simulink model "TestSetup"  (R2022a)
settings: Solver=VariableStepAuto  StartTime=0.0  StopTime=10.0  RelTol=1e-3
undefined symbols (not defined in the file or in its folder): ignition_1, ignition_2, ignition_3, ignition_4, ignition_dwell_time, injection_duration, injection_start_1, injection_start_2, injection_start_3, injection_start_4
libraries: simulink x10
settings Model: Creator=feyzi  LastModifiedBy=feyzi

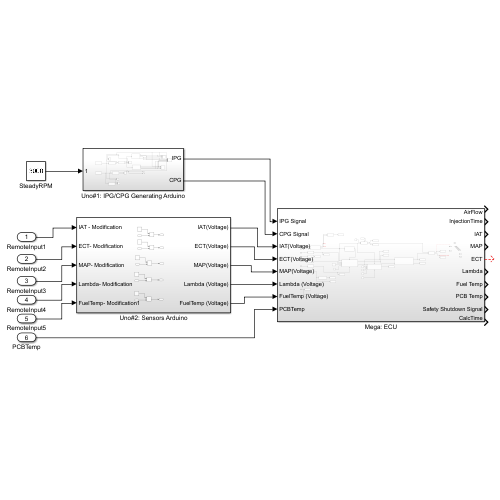
[thumbnail: Simulink's stored preview of the top-level diagram]
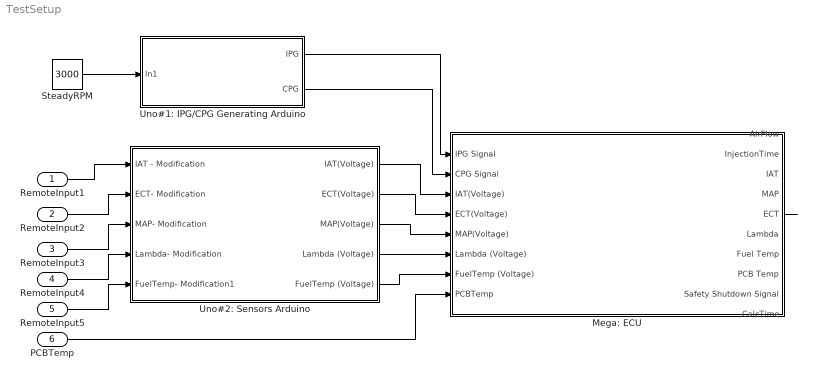
== system TestSetup ==
  RemoteInput1 : Inport
  RemoteInput2 : Inport  Port=2
  RemoteInput3 : Inport  Port=3
  RemoteInput4 : Inport  Port=4
  RemoteInput5 : Inport  Port=5
  PCBTemp : Inport  Port=6
  Mega: ECU : Subsystem
  SteadyRPM : Constant  Value=3000
  Uno#1: IPG/CPG Generating Arduino : Subsystem
  Uno#2: Sensors Arduino : Subsystem
  wires:
  RemoteInput1/1 -> Uno#2: Sensors Arduino/1(IAT - Modification)
  RemoteInput2/1 -> Uno#2: Sensors Arduino/2(ECT- Modification)
  RemoteInput3/1 -> Uno#2: Sensors Arduino/3(MAP- Modification)
  RemoteInput4/1 -> Uno#2: Sensors Arduino/4(Lambda- Modification)
  RemoteInput5/1 -> Uno#2: Sensors Arduino/5(FuelTemp- Modification1)
  Uno#2: Sensors Arduino/1(IAT(Voltage)) -> Mega: ECU/3(IAT(Voltage))
  Uno#2: Sensors Arduino/2(ECT(Voltage)) -> Mega: ECU/4(ECT(Voltage))
  Uno#2: Sensors Arduino/3(MAP(Voltage)) -> Mega: ECU/5(MAP(Voltage))
  Uno#2: Sensors Arduino/4(Lambda (Voltage)) -> Mega: ECU/6(Lambda (Voltage))
  Uno#2: Sensors Arduino/5(FuelTemp (Voltage)) -> Mega: ECU/7(FuelTemp (Voltage))
  PCBTemp/1 -> Mega: ECU/8(PCBTemp)
  SteadyRPM/1 -> Uno#1: IPG/CPG Generating Arduino/1(In1)
  Uno#1: IPG/CPG Generating Arduino/1(IPG) -> Mega: ECU/1(IPG Signal)
  Uno#1: IPG/CPG Generating Arduino/2(CPG) -> Mega: ECU/2(CPG Signal)
  Mega: ECU/5(ECT) -> ?

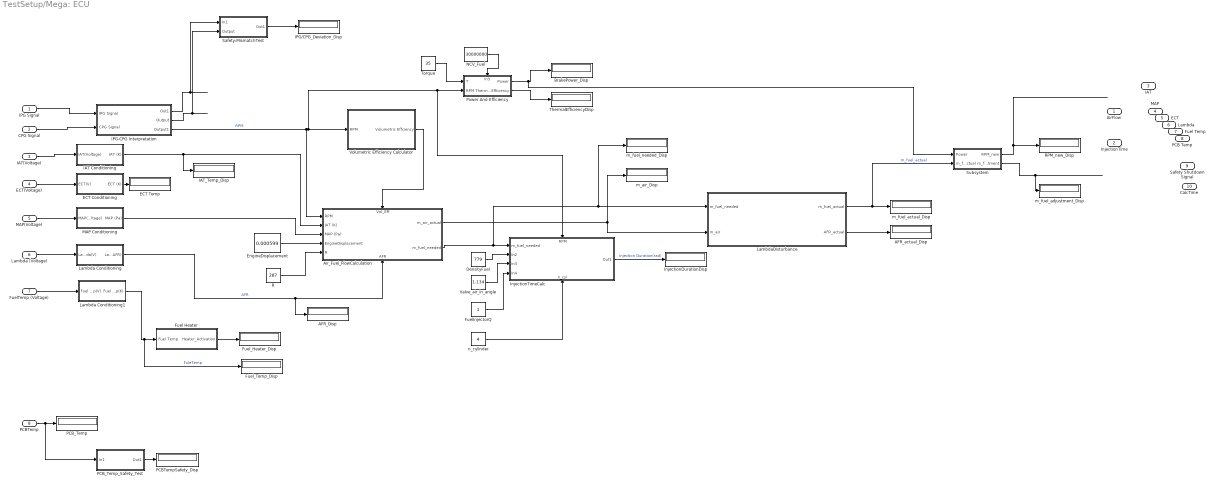
== system TestSetup/Mega: ECU ==
  IPG Signal : Inport
  CPG Signal : Inport  Port=2
  IAT(Voltage) : Inport  Port=3
  ECT(Voltage) : Inport  Port=4
  MAP(Voltage) : Inport  Port=5
  Lambda (Voltage) : Inport  Port=6
  FuelTemp (Voltage) : Inport  Port=7
  PCBTemp : Inport  Port=8
  AFR_Disp : Display
  AFR_actual_Disp : Display
  Air_Fuel_FlowCalculation : Subsystem
      settings: PortSchema="{\"entries\":[{\"content\":{\"sides\":[{\"content\":{\"connectorIds\":[\"In1\",\"In2\",\"In3\",\"In4\",\"In5\"]},\"type\":\"ConnectorPlacement.EquallySpacedRectSide\",\"uuid\":\"ac837b3a-3299-4579-a5f4-28e6eceafe2a\"},{\"content\":{\"connectorIds\":[\"Out1\",\"Out2\"],\"side\":\"RIGHT\"},\"type\":\"ConnectorPlacement.EquallySpacedRectSide\",\"uuid\":\"e1859a27-830c-4dac-bb73-ceffea8c29ce\"},{\"content\":{\"connectorIds\":[\"In6\"],\"side\":\"TOP\"},\"type\":\"ConnectorPlacement.EquallySpacedRectSide\",\"uuid\":\"f305f5bf-787a-4635-84c9-c02b37e24355\"},{\"content\":{\"connectorIds\":[\"In7\"],\"side\":\"BOTTOM\"},\"type\":\"ConnectorPlacement.EquallySpacedRectSide\",\"uuid\":\"b9c30ef4-a18f-4d96-bb00-033b4f03e588\"}]},\"type\":\"ConnectorPlacement.EquallySpacedConnector\",\"uuid\":\"e7c7efd2-9f43-49ae-a3b2-9ba67b40aa2d\"}],\"packageUris\":[\"http://schema.mathworks.com/mf0/Connector/R2020b\"],\"version\":\"1.0\"}"
  BrakePower_Disp : Display
  DensityFuel : Constant  Value=779
  ECT Conditioning : Subsystem
  ECT Temp : Display
  EngineDisplacement : Constant  Value=0.000599
  Fuel Heater : Subsystem
  FuelInjectorQ : Constant
  Fuel_Heater_Disp : Display
  Fuel_Temp_Disp : Display
  IAT Conditioning : Subsystem
  IAT_Temp_Disp : Display
  IPG-CPG Interpretation : Subsystem
  IPG/CPG_Deviation_Disp : Display
  InjectionDurationDisp : Display
  InjectionTimeCalc : Subsystem
      settings: PortSchema="{\"entries\":[{\"content\":{\"sides\":[{\"content\":{\"connectorIds\":[\"In1\",\"In2\",\"In3\",\"In4\"]},\"type\":\"ConnectorPlacement.EquallySpacedRectSide\",\"uuid\":\"ebdf0fa4-cc98-4ade-83ad-774b40e50e14\"},{\"content\":{\"connectorIds\":[\"Out1\"],\"side\":\"RIGHT\"},\"type\":\"ConnectorPlacement.EquallySpacedRectSide\",\"uuid\":\"8b1fcbdc-dea4-4525-97e7-1c674fd2a011\"},{\"content\":{\"connectorIds\":[\"In5\"],\"side\":\"TOP\"},\"type\":\"ConnectorPlacement.EquallySpacedRectSide\",\"uuid\":\"e38dc828-2b63-47c7-a128-8e05c6a6408b\"},{\"content\":{\"connectorIds\":[\"In6\"],\"side\":\"BOTTOM\"},\"type\":\"ConnectorPlacement.EquallySpacedRectSide\",\"uuid\":\"af069764-e087-4372-a960-1041a53fa6fc\"}]},\"type\":\"ConnectorPlacement.EquallySpacedConnector\",\"uuid\":\"8f444e95-b70b-4e07-afd3-af5c44a892f3\"}],\"packageUris\":[\"http://schema.mathworks.com/mf0/Connector/R2020b\"],\"version\":\"1.0\"}"
  Lambda Conditioning : Subsystem
  Lambda Conditioning1 : Subsystem
  LambdaDisturbance : Subsystem
  MAP Conditioning : Subsystem
  NCV_Fuel : Constant  Value=30000000
  PCBTempSafety_Disp : Display
  PCB_Temp : Display
  PCB_Temp_Safety_Test : Subsystem
  Power And Efficiency : Subsystem
      settings: PortSchema="{\"entries\":[{\"content\":{\"sides\":[{\"content\":{\"connectorIds\":[\"In1\",\"In2\"]},\"type\":\"ConnectorPlacement.EquallySpacedRectSide\",\"uuid\":\"acf79f69-6a10-44e4-b57d-bca1c6d4b241\"},{\"content\":{\"connectorIds\":[\"Out1\",\"Out2\"],\"side\":\"RIGHT\"},\"type\":\"ConnectorPlacement.EquallySpacedRectSide\",\"uuid\":\"336ed026-27e8-4de6-8253-c2a43c0fc710\"},{\"content\":{\"connectorIds\":[\"In3\"],\"side\":\"TOP\"},\"type\":\"ConnectorPlacement.EquallySpacedRectSide\",\"uuid\":\"3ecf9081-b2cf-495d-8221-6fb78c14c58c\"}]},\"type\":\"ConnectorPlacement.EquallySpacedConnector\",\"uuid\":\"3fda077c-3971-4965-af51-7420bd2b8db3\"}],\"packageUris\":[\"http://schema.mathworks.com/mf0/Connector/R2020b\"],\"version\":\"1.0\"}"
  R : Constant  Value=287
  RPM_new_Disp : Display
  Safety:MismatchTest : Subsystem
  Subsystem : Subsystem
  ThermalEfficiencyDisp : Display
  Torque : Constant  Value=35
  Valve_air_in_angle : Constant  Value=1.134
  Volumetric Efficiency Calculator : Subsystem
  m_air_Disp : Display
  m_fuel_actual_Disp : Display
  m_fuel_adjustment_Disp : Display
  m_fuel_needed_Disp : Display
  n_cylinder : Constant  Value=4
  AirFlow : Outport
  InjectionTime : Outport  Port=2
  IAT : Outport  Port=3
  MAP : Outport  Port=4
  ECT : Outport  Port=5
  Lambda : Outport  Port=6
  Fuel Temp : Outport  Port=7
  PCB Temp : Outport  Port=8
  Safety Shutdown Signal : Outport  Port=9
  CalcTime : Outport  Port=10
  wires:
  IPG Signal/1 -> IPG-CPG Interpretation/1(IPG Signal)
  CPG Signal/1 -> IPG-CPG Interpretation/2(CPG Signal)
  IPG-CPG Interpretation/1(Out1) -> Safety:MismatchTest/1(In1)
  IPG-CPG Interpretation/2(Output) -> Safety:MismatchTest/2(Output)
  ECT(Voltage)/1 -> ECT Conditioning/1(ECT(V))
  ECT Conditioning/1(ECT (K)) -> ECT Temp/1
  IAT(Voltage)/1 -> IAT Conditioning/1(IAT(Voltage))
  MAP(Voltage)/1 -> MAP Conditioning/1(MAP(Voltage))
  MAP Conditioning/1(MAP (Pa)) -> Air_Fuel_FlowCalculation/3(MAP (Pa))
  Lambda (Voltage)/1 -> Lambda Conditioning/1(Lambda(V))
  FuelTemp (Voltage)/1 -> Lambda Conditioning1/1(Fuel Temp(V))
  Volumetric Efficiency Calculator/1(Volumetric Effciency) -> Air_Fuel_FlowCalculation/6(Vol_Eff)
  EngineDisplacement/1 -> Air_Fuel_FlowCalculation/4(EngineDisplacement)
  R/1 -> Air_Fuel_FlowCalculation/5(R)
  IPG-CPG Interpretation/3(Output1) -> Air_Fuel_FlowCalculation/1(RPM), InjectionTimeCalc/5(RPM), Power And Efficiency/2(RPM), Volumetric Efficiency Calculator/1(RPM)  "RPM"
  IAT Conditioning/1(IAT (K)) -> IAT_Temp_Disp/1, Air_Fuel_FlowCalculation/2(IAT (K))
  Air_Fuel_FlowCalculation/1(m_air_actual) -> m_air_Disp/1, LambdaDisturbance/2(m_air)
  Torque/1 -> Power And Efficiency/1(T)
  Lambda Conditioning1/1(Fuel Temp(K)) -> Fuel_Temp_Disp/1, Fuel Heater/1(Fuel Temp)  "FuleTemp"
  Fuel Heater/1(Heater_Activation) -> Fuel_Heater_Disp/1
  Lambda Conditioning/1(Lambda(AFR)) -> AFR_Disp/1, Air_Fuel_FlowCalculation/7(AFR)  "AFR"
  Air_Fuel_FlowCalculation/2(m_fuel_needed) -> m_fuel_needed_Disp/1, LambdaDisturbance/1(m_fuel_needed), InjectionTimeCalc/1(m_fuel_needed)
  DensityFuel/1 -> InjectionTimeCalc/2(In2)
  Valve_air_in_angle/1 -> InjectionTimeCalc/3(In3)
  NCV_Fuel/1 -> Power And Efficiency/3(In3)
  FuelInjectorQ/1 -> InjectionTimeCalc/4(In4)
  InjectionTimeCalc/1(Out1) -> InjectionDurationDisp/1  "Injection Duration(rad)"
  LambdaDisturbance/1(m_fuel_actual) -> Subsystem/2(m_fuel_actual), m_fuel_actual_Disp/1  "m_fuel_actual"
  LambdaDisturbance/2(AFR_actual) -> AFR_actual_Disp/1
  Power And Efficiency/1(Power) -> Subsystem/1(Power), BrakePower_Disp/1
  Power And Efficiency/2(ThermalEfficiency) -> ThermalEfficiencyDisp/1
  n_cylinder/1 -> InjectionTimeCalc/6(n_cyl)
  Subsystem/1(RPM_new) -> RPM_new_Disp/1
  Subsystem/2(m_fuel_adjustment) -> m_fuel_adjustment_Disp/1
  Safety:MismatchTest/1(Out1) -> IPG/CPG_Deviation_Disp/1
  PCBTemp/1 -> PCB_Temp_Safety_Test/1(In1), PCB_Temp/1
  PCB_Temp_Safety_Test/1(Out1) -> PCBTempSafety_Disp/1

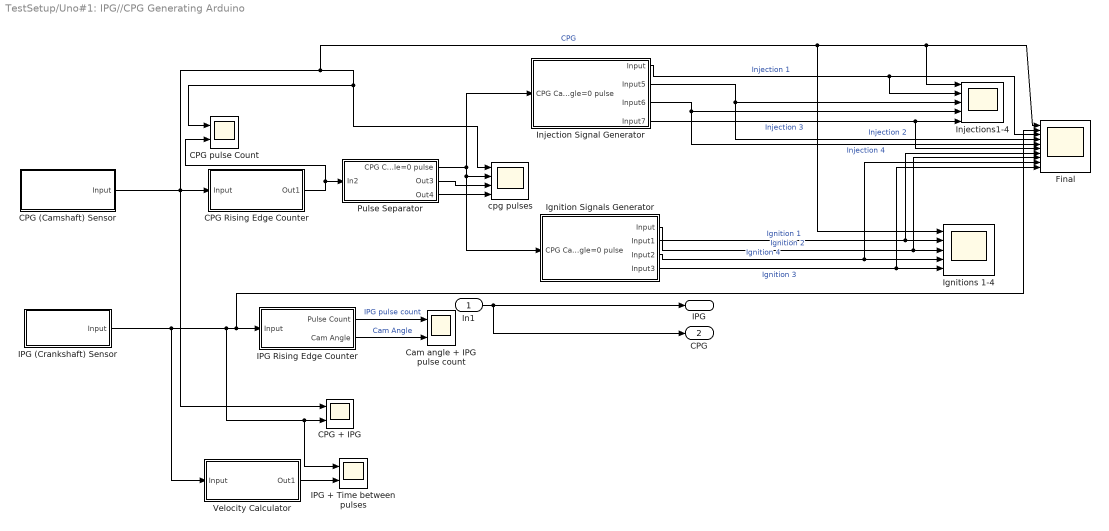
== system TestSetup/Uno#1: IPG//CPG Generating Arduino ==
  In1 : Inport
  CPG (Camshaft) Sensor : Subsystem
  CPG + IPG : Scope  NumInputPorts=2
  CPG Rising Edge Counter : Subsystem
  CPG pulse Count : Scope  NumInputPorts=2
  Cam angle + IPG pulse count : Scope  NumInputPorts=2
  Final : Scope  NumInputPorts=10
  IPG (Crankshaft) Sensor : Subsystem
  IPG + Time between pulses : Scope  NumInputPorts=2
  IPG Rising Edge Counter : Subsystem
  Ignition Signals Generator : Subsystem
  Ignitions 1-4 : Scope  NumInputPorts=5
  Injection Signal Generator : Subsystem
  Injections1-4 : Scope  NumInputPorts=5
  Pulse Separator : Subsystem
  Velocity Calculator : Subsystem
  cpg pulses : Scope  NumInputPorts=4
  IPG : Outport
  CPG : Outport  Port=2
  wires:
  In1/1 -> CPG/1, IPG/1
  IPG Rising Edge Counter/2(Cam Angle) -> Cam angle + IPG pulse count/2  "Cam Angle"
  IPG Rising Edge Counter/1(Pulse Count) -> Cam angle + IPG pulse count/1  "IPG pulse count"
  CPG Rising Edge Counter/1(Out1) -> Pulse Separator/1(In2), CPG pulse Count/2
  Velocity Calculator/1(Out1) -> IPG + Time between pulses/2
  Injection Signal Generator/1(Input) -> Injections1-4/2, Final/3  "Injection 1"
  Ignition Signals Generator/3(Input2) -> Final/9, Ignitions 1-4/4  "Ignition 4"
  Ignition Signals Generator/2(Input1) -> Final/8, Ignitions 1-4/3  "Ignition 2"
  Ignition Signals Generator/1(Input) -> Final/7, Ignitions 1-4/2  "Ignition 1"
  Injection Signal Generator/3(Input6) -> Final/5, Injections1-4/4  "Injection 4"
  Ignition Signals Generator/4(Input3) -> Final/10, Ignitions 1-4/5  "Ignition 3"
  IPG (Crankshaft) Sensor/1(Input) -> IPG Rising Edge Counter/1(Input), Final/2, CPG + IPG/2, IPG + Time between pulses/1, Velocity Calculator/1(Input)
  CPG (Camshaft) Sensor/1(Input) -> Final/1, Injections1-4/1, Ignitions 1-4/1, cpg pulses/1, CPG pulse Count/1, CPG Rising Edge Counter/1(Input), CPG + IPG/1  "CPG"
  Injection Signal Generator/4(Input7) -> Injections1-4/5, Final/6  "Injection 3"
  Pulse Separator/2(Out3) -> cpg pulses/3
  Pulse Separator/3(Out4) -> cpg pulses/4
  Injection Signal Generator/2(Input5) -> Injections1-4/3, Final/4  "Injection 2"
  Pulse Separator/1(CPG Cam Angle=0 pulse) -> Ignition Signals Generator/1(CPG Cam Angle=0 pulse), cpg pulses/2, Injection Signal Generator/1(CPG Cam Angle=0 pulse)

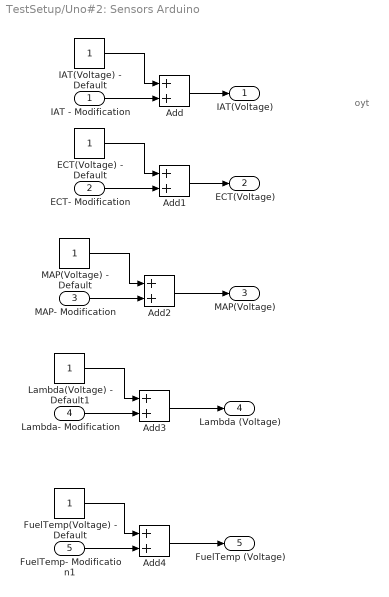
== system TestSetup/Uno#2: Sensors Arduino ==
  note: oyt
  IAT - Modification : Inport
  ECT- Modification : Inport  Port=2
  MAP- Modification : Inport  Port=3
  Lambda- Modification : Inport  Port=4
  FuelTemp- Modification1 : Inport  Port=5
  Add{,1..4} (5 alike) : Sum
  ECT(Voltage) - Default : Constant
  FuelTemp(Voltage) - Default : Constant
  IAT(Voltage) - Default : Constant
  Lambda(Voltage) - Default1 : Constant
  MAP(Voltage) - Default : Constant
  IAT(Voltage) : Outport
  ECT(Voltage) : Outport  Port=2
  MAP(Voltage) : Outport  Port=3
  Lambda (Voltage) : Outport  Port=4
  FuelTemp (Voltage) : Outport  Port=5
  wires:
  IAT(Voltage) - Default/1 -> Add/1
  IAT - Modification/1 -> Add/2
  Add/1 -> IAT(Voltage)/1
  ECT- Modification/1 -> Add1/2
  ECT(Voltage) - Default/1 -> Add1/1
  Add1/1 -> ECT(Voltage)/1
  MAP(Voltage) - Default/1 -> Add2/1
  MAP- Modification/1 -> Add2/2
  Lambda- Modification/1 -> Add3/2
  Lambda(Voltage) - Default1/1 -> Add3/1
  Add2/1 -> MAP(Voltage)/1
  Add3/1 -> Lambda (Voltage)/1
  FuelTemp(Voltage) - Default/1 -> Add4/1
  FuelTemp- Modification1/1 -> Add4/2
  Add4/1 -> FuelTemp (Voltage)/1

== system TestSetup/Mega: ECU/Air_Fuel_FlowCalculation ==
  RPM : Inport
  IAT (K) : Inport  Port=2
  MAP (Pa) : Inport  Port=3
  EngineDisplacement : Inport  Port=4
  R : Inport  Port=5
  Vol_Eff : Inport  Port=6
  AFR : Inport  Port=7
  m_air_actual : Outport
  m_fuel_needed : Outport  Port=2
  wires:
  MAP (Pa)/1 -> m_air_actual/1

== system TestSetup/Mega: ECU/ECT Conditioning ==
  ECT(V) : Inport
  ECT (K) : Outport
  wires:
  ECT(V)/1 -> ECT (K)/1

== system TestSetup/Mega: ECU/Fuel Heater ==
  Fuel Temp : Inport
  Heater_Activation : Outport
  wires:
  Fuel Temp/1 -> Heater_Activation/1

== system TestSetup/Mega: ECU/IAT Conditioning ==
  IAT(Voltage) : Inport
  IAT (K) : Outport
  wires:
  IAT(Voltage)/1 -> IAT (K)/1

== system TestSetup/Mega: ECU/IPG-CPG Interpretation ==
  IPG Signal : Inport
  CPG Signal : Inport  Port=2
  Out1 : Outport
  Output : Outport  Port=2
  Output1 : Outport  Port=3
  wires:
  IPG Signal/1 -> Out1/1
  CPG Signal/1 -> Output/1

== system TestSetup/Mega: ECU/InjectionTimeCalc ==
  m_fuel_needed : Inport
  In2 : Inport  Port=2
  In3 : Inport  Port=3
  In4 : Inport  Port=4
  RPM : Inport  Port=5
  n_cyl : Inport  Port=6
  Out1 : Outport
  wires:
  m_fuel_needed/1 -> Out1/1

== system TestSetup/Mega: ECU/Lambda Conditioning ==
  Lambda(V) : Inport
  Lambda(AFR) : Outport
  wires:
  Lambda(V)/1 -> Lambda(AFR)/1

== system TestSetup/Mega: ECU/Lambda Conditioning1 ==
  Fuel Temp(V) : Inport
  Fuel Temp(K) : Outport
  wires:
  Fuel Temp(V)/1 -> Fuel Temp(K)/1

== system TestSetup/Mega: ECU/LambdaDisturbance ==
  m_fuel_needed : Inport
  m_air : Inport  Port=2
  m_fuel_actual : Outport
  AFR_actual : Outport  Port=2
  wires:
  m_fuel_needed/1 -> m_fuel_actual/1

== system TestSetup/Mega: ECU/MAP Conditioning ==
  MAP(Voltage) : Inport
  MAP (Pa) : Outport
  wires:
  MAP(Voltage)/1 -> MAP (Pa)/1

== system TestSetup/Mega: ECU/PCB_Temp_Safety_Test ==
  In1 : Inport
  Out1 : Outport
  wires:
  In1/1 -> Out1/1

== system TestSetup/Mega: ECU/Power And Efficiency ==
  T : Inport
  RPM : Inport  Port=2
  In3 : Inport  Port=3
  Power : Outport
  ThermalEfficiency : Outport  Port=2
  wires:
  RPM/1 -> Power/1

== system TestSetup/Mega: ECU/Safety:MismatchTest ==
  In1 : Inport
  Output : Inport  Port=2
  Out1 : Outport
  wires:
  In1/1 -> Out1/1

== system TestSetup/Mega: ECU/Subsystem ==
  Power : Inport
  m_fuel_actual : Inport  Port=2
  RPM_new : Outport
  m_fuel_adjustment : Outport  Port=2
  wires:
  Power/1 -> RPM_new/1

== system TestSetup/Mega: ECU/Volumetric Efficiency Calculator ==
  RPM : Inport
  Volumetric Effciency : Outport
  wires:
  RPM/1 -> Volumetric Effciency/1

== system TestSetup/Uno#1: IPG//CPG Generating Arduino/CPG (Camshaft) Sensor ==
  Peak 2(Ref) : DiscretePulseGenerator  PulseType=Time based  Period=1  PulseWidth=5  PhaseDelay=0.1
  Peak 3 (TDC- before Power) : DiscretePulseGenerator  PulseType=Time based  Period=1  PulseWidth=5  PhaseDelay=0.5
  Peak1(cycle start - injection TDC) : DiscretePulseGenerator  PulseType=Time based  Period=1  PulseWidth=5
  Sum : Sum  Inputs=|+++  InputSameDT=on
  Unit Delay1 : UnitDelay  SampleTime=-1  HasFrameUpgradeWarning=on
  Input : Outport
  wires:
  Sum/1 -> Unit Delay1/1
  Peak1(cycle start - injection TDC)/1 -> Sum/1
  Peak 2(Ref)/1 -> Sum/2
  Peak 3 (TDC- before Power)/1 -> Sum/3
  Unit Delay1/1 -> Input/1

== system TestSetup/Uno#1: IPG//CPG Generating Arduino/CPG Rising Edge Counter ==
  Input : Inport
  Count Resetter : simulink/Logic and Bit Operations/Compare To Constant  relop=>=  const=3.0  OutDataTypeStr=boolean
  Delay : Delay  DelayLength=1
  Detect Rise Positive : simulink/Logic and Bit Operations/Detect Rise Positive  vinit=0  OutDataTypeStr=uint8
  Rising Edge Counter : Subsystem  TreatAsAtomicUnit=on
  Scope : Scope  NumInputPorts=2
  Out1 : Outport
  wires:
  Delay/1 -> Rising Edge Counter/Reset
  Input/1 -> Detect Rise Positive/1, Scope/1  "CPG signal"
  Detect Rise Positive/1 -> Rising Edge Counter/1(In1)  "Rising Edge Detected"
  Count Resetter/1 -> Delay/1
  Rising Edge Counter/1(Out1) -> Out1/1, Scope/2, Count Resetter/1  "CPG Pulse Count"

== system TestSetup/Uno#1: IPG//CPG Generating Arduino/IPG (Crankshaft) Sensor ==
  Pulse Generator : DiscretePulseGenerator  PulseType=Time based  Period=0.042  PulseWidth=5
  Input : Outport
  wires:
  Pulse Generator/1 -> Input/1

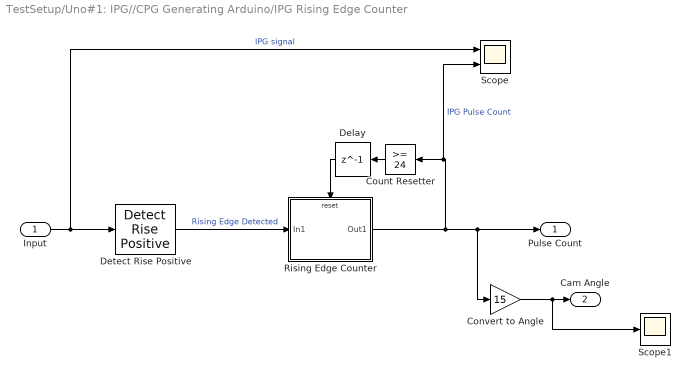
== system TestSetup/Uno#1: IPG//CPG Generating Arduino/IPG Rising Edge Counter ==
  Input : Inport
  Convert to Angle : Gain  Gain=15
  Count Resetter : simulink/Logic and Bit Operations/Compare To Constant  relop=>=  const=24  OutDataTypeStr=boolean
  Delay : Delay  DelayLength=1
  Detect Rise Positive : simulink/Logic and Bit Operations/Detect Rise Positive  vinit=0  OutDataTypeStr=uint8
  Rising Edge Counter : Subsystem  TreatAsAtomicUnit=on
  Scope : Scope  NumInputPorts=2
  Scope1 : Scope
  Pulse Count : Outport
  Cam Angle : Outport  Port=2
  wires:
  Delay/1 -> Rising Edge Counter/Reset
  Input/1 -> Detect Rise Positive/1, Scope/1  "IPG signal"
  Detect Rise Positive/1 -> Rising Edge Counter/1(In1)  "Rising Edge Detected"
  Count Resetter/1 -> Delay/1
  Rising Edge Counter/1(Out1) -> Convert to Angle/1, Pulse Count/1, Scope/2, Count Resetter/1  "IPG Pulse Count"
  Convert to Angle/1 -> Scope1/1, Cam Angle/1

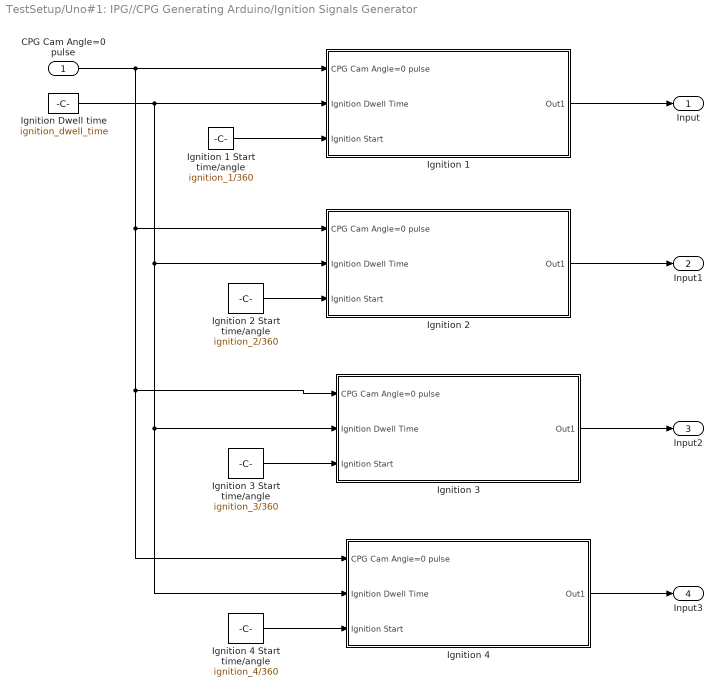
== system TestSetup/Uno#1: IPG//CPG Generating Arduino/Ignition Signals Generator ==
  CPG Cam Angle=0 pulse : Inport
  Ignition 1 : Subsystem
  Ignition 1 Start time/angle : Constant  Value=ignition_1/360
  Ignition 2 : Subsystem
  Ignition 2 Start time/angle : Constant  Value=ignition_2/360
  Ignition 3 : Subsystem
  Ignition 3 Start time/angle : Constant  Value=ignition_3/360
  Ignition 4 : Subsystem
  Ignition 4 Start time/angle : Constant  Value=ignition_4/360
  Ignition Dwell time : Constant  Value=ignition_dwell_time
  Input : Outport
  Input1 : Outport  Port=2
  Input2 : Outport  Port=3
  Input3 : Outport  Port=4
  wires:
  CPG Cam Angle=0 pulse/1 -> Ignition 2/1(CPG Cam Angle=0 pulse), Ignition 4/1(CPG Cam Angle=0 pulse), Ignition 3/1(CPG Cam Angle=0 pulse), Ignition 1/1(CPG Cam Angle=0 pulse)
  Ignition Dwell time/1 -> Ignition 2/2(Ignition Dwell Time), Ignition 4/2(Ignition Dwell Time), Ignition 3/2(Ignition Dwell Time), Ignition 1/2(Ignition Dwell Time)
  Ignition 1 Start time/angle/1 -> Ignition 1/3(Ignition Start)
  Ignition 1/1(Out1) -> Input/1
  Ignition 2/1(Out1) -> Input1/1
  Ignition 3/1(Out1) -> Input2/1
  Ignition 4/1(Out1) -> Input3/1
  Ignition 2 Start time/angle/1 -> Ignition 2/3(Ignition Start)
  Ignition 3 Start time/angle/1 -> Ignition 3/3(Ignition Start)
  Ignition 4 Start time/angle/1 -> Ignition 4/3(Ignition Start)

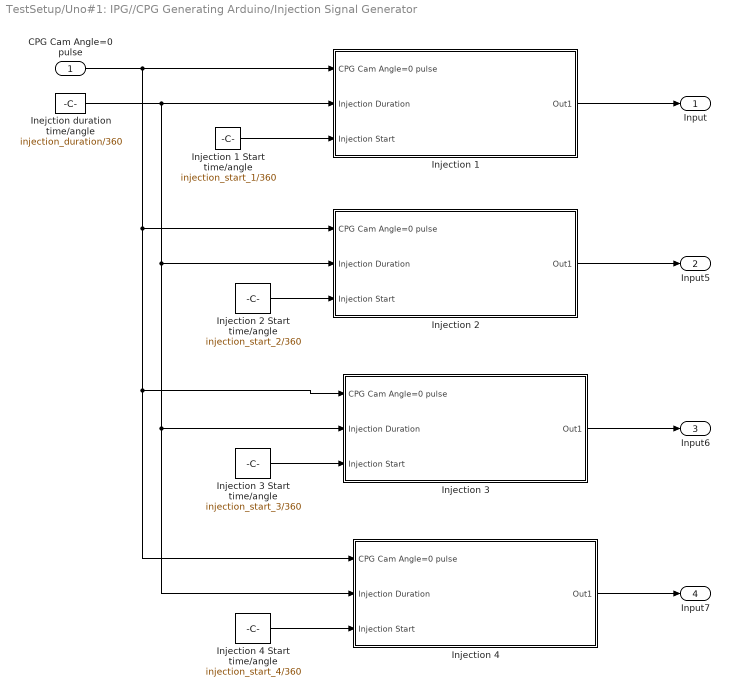
== system TestSetup/Uno#1: IPG//CPG Generating Arduino/Injection Signal Generator ==
  CPG Cam Angle=0 pulse : Inport
  Inejction duration time/angle : Constant  Value=injection_duration/360
  Injection 1 : Subsystem
  Injection 1 Start time/angle : Constant  Value=injection_start_1/360
  Injection 2 : Subsystem
  Injection 2 Start time/angle : Constant  Value=injection_start_2/360
  Injection 3 : Subsystem
  Injection 3 Start time/angle : Constant  Value=injection_start_3/360
  Injection 4 : Subsystem
  Injection 4 Start time/angle : Constant  Value=injection_start_4/360
  Input : Outport
  Input5 : Outport  Port=2
  Input6 : Outport  Port=3
  Input7 : Outport  Port=4
  wires:
  CPG Cam Angle=0 pulse/1 -> Injection 3/1(CPG Cam Angle=0 pulse), Injection 4/1(CPG Cam Angle=0 pulse), Injection 2/1(CPG Cam Angle=0 pulse), Injection 1/1(CPG Cam Angle=0 pulse)
  Inejction duration time/angle/1 -> Injection 4/2(Injection Duration), Injection 3/2(Injection Duration), Injection 2/2(Injection Duration), Injection 1/2(Injection Duration)
  Injection 1 Start time/angle/1 -> Injection 1/3(Injection Start)
  Injection 1/1(Out1) -> Input/1
  Injection 2/1(Out1) -> Input5/1
  Injection 3/1(Out1) -> Input6/1
  Injection 4/1(Out1) -> Input7/1
  Injection 2 Start time/angle/1 -> Injection 2/3(Injection Start)
  Injection 3 Start time/angle/1 -> Injection 3/3(Injection Start)
  Injection 4 Start time/angle/1 -> Injection 4/3(Injection Start)

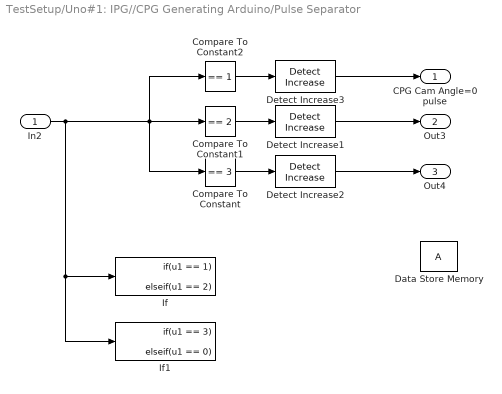
== system TestSetup/Uno#1: IPG//CPG Generating Arduino/Pulse Separator ==
  In2 : Inport
  Compare To Constant : simulink/Logic and Bit Operations/Compare To Constant  relop===  const=3  OutDataTypeStr=uint8
  Compare To Constant1 : simulink/Logic and Bit Operations/Compare To Constant  relop===  const=2  OutDataTypeStr=uint8
  Compare To Constant2 : simulink/Logic and Bit Operations/Compare To Constant  relop===  const=1  OutDataTypeStr=uint8
  Data Store Memory : DataStoreMemory  ReadBeforeWriteMsg=warning  WriteAfterWriteMsg=warning  WriteAfterReadMsg=warning  ShareAcrossModelInstances=on  ShowAdditionalParam=off  OutMin=0  OutMax=12
  Detect Increase1 : simulink/Logic and Bit Operations/Detect Increase  vinit=0.0  OutDataTypeStr=uint8
  Detect Increase2 : simulink/Logic and Bit Operations/Detect Increase  vinit=0.0  OutDataTypeStr=uint8
  Detect Increase3 : simulink/Logic and Bit Operations/Detect Increase  vinit=0.0  OutDataTypeStr=uint8
  If : If  IfExpression=u1 == 1  ElseIfExpressions=u1 == 2  ShowElse=off
  If1 : If  IfExpression=u1 == 3  ElseIfExpressions=u1 == 0  ShowElse=off
  CPG Cam Angle=0 pulse : Outport  OutDataTypeStr=uint8
  Out3 : Outport  Port=2
  Out4 : Outport  Port=3
  wires:
  Detect Increase2/1 -> Out4/1
  In2/1 -> If1/1, If/1, Compare To Constant2/1, Compare To Constant/1, Compare To Constant1/1
  Compare To Constant1/1 -> Detect Increase1/1
  Detect Increase1/1 -> Out3/1
  Compare To Constant/1 -> Detect Increase2/1
  Compare To Constant2/1 -> Detect Increase3/1
  Detect Increase3/1 -> CPG Cam Angle=0 pulse/1

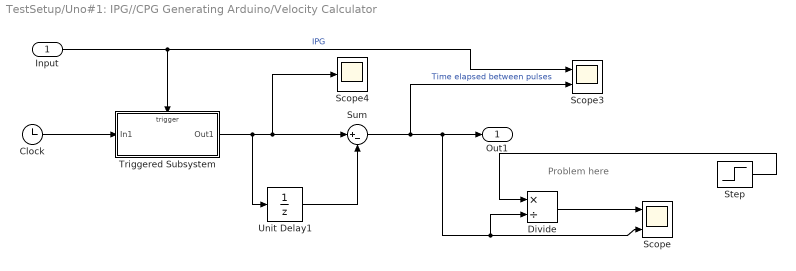
== system TestSetup/Uno#1: IPG//CPG Generating Arduino/Velocity Calculator ==
  note: Problem here
  Input : Inport
  Clock : Clock
      settings: Decimation=100
  Divide : Product  Inputs=*/
  Scope : Scope  NumInputPorts=2
  Scope3 : Scope  NumInputPorts=2
  Scope4 : Scope
  Step : Step  Time=0  After=30/12  SampleTime=0
  Sum : Sum  Inputs=|+-
  Triggered Subsystem : Subsystem  TreatAsAtomicUnit=on
  Unit Delay1 : UnitDelay  SampleTime=-1
  Out1 : Outport
  wires:
  Sum/1 -> Scope3/2, Divide/2, Scope/2, Out1/1  "Time elapsed between pulses"
  Input/1 -> Scope3/1, Triggered Subsystem/Trigger  "IPG"
  Unit Delay1/1 -> Sum/2
  Clock/1 -> Triggered Subsystem/1(In1)
  Triggered Subsystem/1(Out1) -> Sum/1, Scope4/1, Unit Delay1/1
  Step/1 -> Divide/1
  Divide/1 -> Scope/1

== system TestSetup/Uno#1: IPG//CPG Generating Arduino/CPG Rising Edge Counter/Rising Edge Counter ==
  In1 : Inport
  Reset : ResetPort  DisableCoverage=on
  Memory : Memory
  Sum1 : Sum  Inputs=|++
  Out1 : Outport
  wires:
  Memory/1 -> Sum1/2
  Sum1/1 -> Out1/1, Memory/1
  In1/1 -> Sum1/1

== system TestSetup/Uno#1: IPG//CPG Generating Arduino/IPG Rising Edge Counter/Rising Edge Counter ==
  In1 : Inport
  Reset : ResetPort  DisableCoverage=on
  Memory : Memory
  Sum1 : Sum  Inputs=|++
  Out1 : Outport
  wires:
  Memory/1 -> Sum1/2
  Sum1/1 -> Out1/1, Memory/1
  In1/1 -> Sum1/1

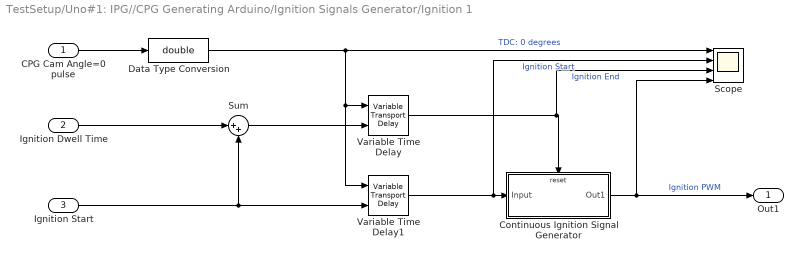
== system TestSetup/Uno#1: IPG//CPG Generating Arduino/Ignition Signals Generator/Ignition 1 ==
  CPG Cam Angle=0 pulse : Inport
  Ignition Dwell Time : Inport  Port=2
  Ignition Start : Inport  Port=3
  Continuous Ignition Signal Generator : Subsystem  TreatAsAtomicUnit=on
  Data Type Conversion : DataTypeConversion  OutDataTypeStr=double  SaturateOnIntegerOverflow=off  RndMeth=Floor
  Scope : Scope  NumInputPorts=4
  Sum : Sum  Inputs=|++
  Variable Time Delay : VariableTransportDelay  MaximumDelay=10  MaximumPoints=20480  ZeroDelay=on
  Variable Time Delay1 : VariableTransportDelay  MaximumDelay=10  MaximumPoints=20480  ZeroDelay=on
  Out1 : Outport
  wires:
  Continuous Ignition Signal Generator/1(Out1) -> Scope/4, Out1/1  "Ignition PWM"
  Variable Time Delay/1 -> Scope/3, Continuous Ignition Signal Generator/Reset  "Ignition End"
  Ignition Start/1 -> Sum/2, Variable Time Delay1/2
  CPG Cam Angle=0 pulse/1 -> Data Type Conversion/1
  Variable Time Delay1/1 -> Scope/2, Continuous Ignition Signal Generator/1(Input)  "Ignition Start"
  Data Type Conversion/1 -> Scope/1, Variable Time Delay1/1, Variable Time Delay/1  "TDC: 0 degrees"
  Ignition Dwell Time/1 -> Sum/1
  Sum/1 -> Variable Time Delay/2

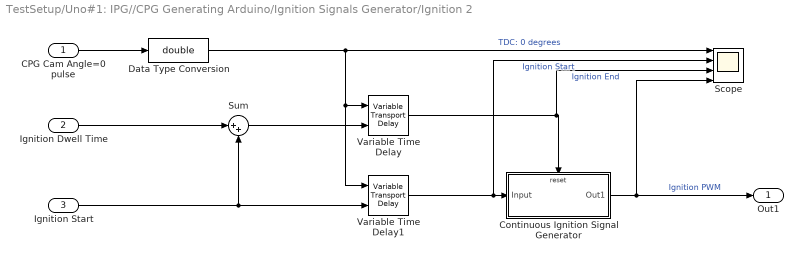
== system TestSetup/Uno#1: IPG//CPG Generating Arduino/Ignition Signals Generator/Ignition 2 ==
  CPG Cam Angle=0 pulse : Inport
  Ignition Dwell Time : Inport  Port=2
  Ignition Start : Inport  Port=3
  Continuous Ignition Signal Generator : Subsystem  TreatAsAtomicUnit=on
  Data Type Conversion : DataTypeConversion  OutDataTypeStr=double  SaturateOnIntegerOverflow=off  RndMeth=Floor
  Scope : Scope  NumInputPorts=4
  Sum : Sum  Inputs=|++
  Variable Time Delay : VariableTransportDelay  MaximumDelay=10  MaximumPoints=20480  ZeroDelay=on
  Variable Time Delay1 : VariableTransportDelay  MaximumDelay=10  MaximumPoints=20480  ZeroDelay=on
  Out1 : Outport
  wires:
  Continuous Ignition Signal Generator/1(Out1) -> Scope/4, Out1/1  "Ignition PWM"
  Variable Time Delay/1 -> Scope/3, Continuous Ignition Signal Generator/Reset  "Ignition End"
  Ignition Start/1 -> Sum/2, Variable Time Delay1/2
  CPG Cam Angle=0 pulse/1 -> Data Type Conversion/1
  Variable Time Delay1/1 -> Scope/2, Continuous Ignition Signal Generator/1(Input)  "Ignition Start"
  Data Type Conversion/1 -> Scope/1, Variable Time Delay1/1, Variable Time Delay/1  "TDC: 0 degrees"
  Ignition Dwell Time/1 -> Sum/1
  Sum/1 -> Variable Time Delay/2

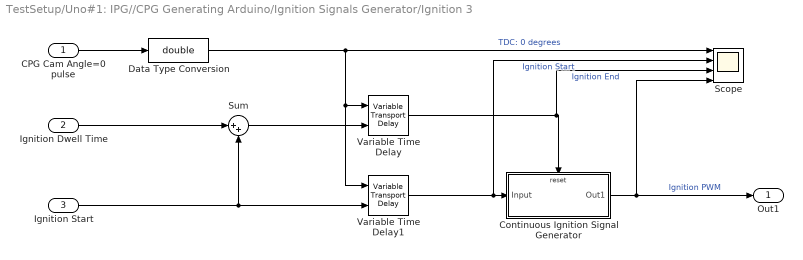
== system TestSetup/Uno#1: IPG//CPG Generating Arduino/Ignition Signals Generator/Ignition 3 ==
  CPG Cam Angle=0 pulse : Inport
  Ignition Dwell Time : Inport  Port=2
  Ignition Start : Inport  Port=3
  Continuous Ignition Signal Generator : Subsystem  TreatAsAtomicUnit=on
  Data Type Conversion : DataTypeConversion  OutDataTypeStr=double  SaturateOnIntegerOverflow=off  RndMeth=Floor
  Scope : Scope  NumInputPorts=4
  Sum : Sum  Inputs=|++
  Variable Time Delay : VariableTransportDelay  MaximumDelay=10  MaximumPoints=20480  ZeroDelay=on
  Variable Time Delay1 : VariableTransportDelay  MaximumDelay=10  MaximumPoints=20480  ZeroDelay=on
  Out1 : Outport
  wires:
  Continuous Ignition Signal Generator/1(Out1) -> Scope/4, Out1/1  "Ignition PWM"
  Variable Time Delay/1 -> Scope/3, Continuous Ignition Signal Generator/Reset  "Ignition End"
  Ignition Start/1 -> Sum/2, Variable Time Delay1/2
  CPG Cam Angle=0 pulse/1 -> Data Type Conversion/1
  Variable Time Delay1/1 -> Scope/2, Continuous Ignition Signal Generator/1(Input)  "Ignition Start"
  Data Type Conversion/1 -> Scope/1, Variable Time Delay1/1, Variable Time Delay/1  "TDC: 0 degrees"
  Ignition Dwell Time/1 -> Sum/1
  Sum/1 -> Variable Time Delay/2

== system TestSetup/Uno#1: IPG//CPG Generating Arduino/Ignition Signals Generator/Ignition 4 ==
  CPG Cam Angle=0 pulse : Inport
  Ignition Dwell Time : Inport  Port=2
  Ignition Start : Inport  Port=3
  Continuous Ignition Signal Generator : Subsystem  TreatAsAtomicUnit=on
  Data Type Conversion : DataTypeConversion  OutDataTypeStr=double  SaturateOnIntegerOverflow=off  RndMeth=Floor
  Scope : Scope  NumInputPorts=4
  Sum : Sum  Inputs=|++
  Variable Time Delay : VariableTransportDelay  MaximumDelay=10  MaximumPoints=20480  ZeroDelay=on
  Variable Time Delay1 : VariableTransportDelay  MaximumDelay=10  MaximumPoints=20480  ZeroDelay=on
  Out1 : Outport
  wires:
  Continuous Ignition Signal Generator/1(Out1) -> Scope/4, Out1/1  "Ignition PWM"
  Variable Time Delay/1 -> Scope/3, Continuous Ignition Signal Generator/Reset  "Ignition End"
  Ignition Start/1 -> Variable Time Delay1/2, Sum/2
  CPG Cam Angle=0 pulse/1 -> Data Type Conversion/1
  Variable Time Delay1/1 -> Scope/2, Continuous Ignition Signal Generator/1(Input)  "Ignition Start"
  Data Type Conversion/1 -> Scope/1, Variable Time Delay1/1, Variable Time Delay/1  "TDC: 0 degrees"
  Ignition Dwell Time/1 -> Sum/1
  Sum/1 -> Variable Time Delay/2

== system TestSetup/Uno#1: IPG//CPG Generating Arduino/Injection Signal Generator/Injection 1 ==
  CPG Cam Angle=0 pulse : Inport
  Injection Duration : Inport  Port=2
  Injection Start : Inport  Port=3
  Continuous Injection Signal Generator : Subsystem  TreatAsAtomicUnit=on
  Data Type Conversion : DataTypeConversion  OutDataTypeStr=double  SaturateOnIntegerOverflow=off  RndMeth=Floor
  Scope : Scope  NumInputPorts=4
  Sum : Sum  Inputs=|++
  Variable Time Delay : VariableTransportDelay  MaximumDelay=10  MaximumPoints=20480  ZeroDelay=on
  Variable Time Delay1 : VariableTransportDelay  MaximumDelay=10  MaximumPoints=30720  ZeroDelay=on
  Out1 : Outport
  wires:
  Continuous Injection Signal Generator/1(Out1) -> Scope/4, Out1/1  "Injection 1 pwm"
  Variable Time Delay/1 -> Scope/3, Continuous Injection Signal Generator/Reset  "Injection 1 end"
  Injection Start/1 -> Sum/2, Variable Time Delay1/2
  CPG Cam Angle=0 pulse/1 -> Data Type Conversion/1
  Variable Time Delay1/1 -> Scope/2, Continuous Injection Signal Generator/1(Input)  "Injection 1 start"
  Data Type Conversion/1 -> Scope/1, Variable Time Delay1/1, Variable Time Delay/1  "TDC: 0 degrees"
  Injection Duration/1 -> Sum/1
  Sum/1 -> Variable Time Delay/2

== system TestSetup/Uno#1: IPG//CPG Generating Arduino/Injection Signal Generator/Injection 2 ==
  CPG Cam Angle=0 pulse : Inport
  Injection Duration : Inport  Port=2
  Injection Start : Inport  Port=3
  Continuous Injection Signal Generator : Subsystem  TreatAsAtomicUnit=on
  Data Type Conversion : DataTypeConversion  OutDataTypeStr=double  SaturateOnIntegerOverflow=off  RndMeth=Floor
  Scope : Scope  NumInputPorts=4
  Sum : Sum  Inputs=|++
  Variable Time Delay : VariableTransportDelay  MaximumDelay=10  MaximumPoints=20480  ZeroDelay=on
  Variable Time Delay1 : VariableTransportDelay  MaximumDelay=10  MaximumPoints=30720  ZeroDelay=on
  Out1 : Outport
  wires:
  Continuous Injection Signal Generator/1(Out1) -> Scope/4, Out1/1  "Injection 2 pwm"
  Variable Time Delay/1 -> Scope/3, Continuous Injection Signal Generator/Reset  "Injection 2 end"
  Injection Start/1 -> Sum/2, Variable Time Delay1/2
  CPG Cam Angle=0 pulse/1 -> Data Type Conversion/1
  Variable Time Delay1/1 -> Scope/2, Continuous Injection Signal Generator/1(Input)  "Injection 2 start"
  Data Type Conversion/1 -> Scope/1, Variable Time Delay1/1, Variable Time Delay/1  "TDC: 0 degrees"
  Injection Duration/1 -> Sum/1
  Sum/1 -> Variable Time Delay/2

== system TestSetup/Uno#1: IPG//CPG Generating Arduino/Injection Signal Generator/Injection 3 ==
  CPG Cam Angle=0 pulse : Inport
  Injection Duration : Inport  Port=2
  Injection Start : Inport  Port=3
  Continuous Injection Signal Generator : Subsystem  TreatAsAtomicUnit=on
  Data Type Conversion : DataTypeConversion  OutDataTypeStr=double  SaturateOnIntegerOverflow=off  RndMeth=Floor
  Scope : Scope  NumInputPorts=4
  Sum : Sum  Inputs=|++
  Variable Time Delay : VariableTransportDelay  MaximumDelay=10  MaximumPoints=20480  ZeroDelay=on
  Variable Time Delay1 : VariableTransportDelay  MaximumDelay=10  MaximumPoints=20480  ZeroDelay=on
  Out1 : Outport
  wires:
  Continuous Injection Signal Generator/1(Out1) -> Scope/4, Out1/1  "Injection 3 pwm"
  Variable Time Delay/1 -> Scope/3, Continuous Injection Signal Generator/Reset  "Injection 3 end"
  Injection Start/1 -> Sum/2, Variable Time Delay1/2
  CPG Cam Angle=0 pulse/1 -> Data Type Conversion/1
  Variable Time Delay1/1 -> Scope/2, Continuous Injection Signal Generator/1(Input)  "Injection 3 start"
  Data Type Conversion/1 -> Scope/1, Variable Time Delay1/1, Variable Time Delay/1  "TDC: 0 degrees"
  Injection Duration/1 -> Sum/1
  Sum/1 -> Variable Time Delay/2

== system TestSetup/Uno#1: IPG//CPG Generating Arduino/Injection Signal Generator/Injection 4 ==
  CPG Cam Angle=0 pulse : Inport
  Injection Duration : Inport  Port=2
  Injection Start : Inport  Port=3
  Continuous Injection Signal Generator : Subsystem  TreatAsAtomicUnit=on
  Data Type Conversion : DataTypeConversion  OutDataTypeStr=double  SaturateOnIntegerOverflow=off  RndMeth=Floor
  Scope : Scope  NumInputPorts=4
  Sum : Sum  Inputs=|++
  Variable Time Delay : VariableTransportDelay  MaximumDelay=10  MaximumPoints=20480  ZeroDelay=on
  Variable Time Delay1 : VariableTransportDelay  MaximumDelay=10  MaximumPoints=20480  ZeroDelay=on
  Out1 : Outport
  wires:
  Continuous Injection Signal Generator/1(Out1) -> Scope/4, Out1/1  "Injection 4 pwm"
  Variable Time Delay/1 -> Scope/3, Continuous Injection Signal Generator/Reset  "Injection 4 end"
  Injection Start/1 -> Sum/2, Variable Time Delay1/2
  CPG Cam Angle=0 pulse/1 -> Data Type Conversion/1
  Variable Time Delay1/1 -> Scope/2, Continuous Injection Signal Generator/1(Input)  "Injection 4 start"
  Data Type Conversion/1 -> Scope/1, Variable Time Delay1/1, Variable Time Delay/1  "TDC: 0 degrees"
  Injection Duration/1 -> Sum/1
  Sum/1 -> Variable Time Delay/2

== system TestSetup/Uno#1: IPG//CPG Generating Arduino/Velocity Calculator/Triggered Subsystem ==
  In1 : Inport
  Trigger : TriggerPort  VariantControl=(inherit)
  Out1 : Outport
  wires:
  In1/1 -> Out1/1

== system TestSetup/Uno#1: IPG//CPG Generating Arduino/Ignition Signals Generator/Ignition 1/Continuous Ignition Signal Generator ==
  Input : Inport
  Reset : ResetPort  DisableCoverage=on
  Memory1 : Memory
  Sum1 : Sum  Inputs=|++
  Out1 : Outport
  wires:
  Sum1/1 -> Out1/1, Memory1/1
  Input/1 -> Sum1/1
  Memory1/1 -> Sum1/2

== system TestSetup/Uno#1: IPG//CPG Generating Arduino/Ignition Signals Generator/Ignition 2/Continuous Ignition Signal Generator ==
  Input : Inport
  Reset : ResetPort  DisableCoverage=on
  Memory1 : Memory
  Sum1 : Sum  Inputs=|++
  Out1 : Outport
  wires:
  Sum1/1 -> Out1/1, Memory1/1
  Input/1 -> Sum1/1
  Memory1/1 -> Sum1/2

== system TestSetup/Uno#1: IPG//CPG Generating Arduino/Ignition Signals Generator/Ignition 3/Continuous Ignition Signal Generator ==
  Input : Inport
  Reset : ResetPort  DisableCoverage=on
  Memory1 : Memory
  Sum1 : Sum  Inputs=|++
  Out1 : Outport
  wires:
  Sum1/1 -> Out1/1, Memory1/1
  Input/1 -> Sum1/1
  Memory1/1 -> Sum1/2

== system TestSetup/Uno#1: IPG//CPG Generating Arduino/Ignition Signals Generator/Ignition 4/Continuous Ignition Signal Generator ==
  Input : Inport
  Reset : ResetPort  DisableCoverage=on
  Memory1 : Memory
  Sum1 : Sum  Inputs=|++
  Out1 : Outport
  wires:
  Sum1/1 -> Out1/1, Memory1/1
  Input/1 -> Sum1/1
  Memory1/1 -> Sum1/2

== system TestSetup/Uno#1: IPG//CPG Generating Arduino/Injection Signal Generator/Injection 1/Continuous Injection Signal Generator ==
  Input : Inport
  Reset : ResetPort  DisableCoverage=on
  Memory1 : Memory
  Sum1 : Sum  Inputs=|++
  Out1 : Outport
  wires:
  Sum1/1 -> Out1/1, Memory1/1
  Input/1 -> Sum1/1
  Memory1/1 -> Sum1/2

== system TestSetup/Uno#1: IPG//CPG Generating Arduino/Injection Signal Generator/Injection 2/Continuous Injection Signal Generator ==
  Input : Inport
  Reset : ResetPort  DisableCoverage=on
  Memory1 : Memory
  Sum1 : Sum  Inputs=|++
  Out1 : Outport
  wires:
  Sum1/1 -> Out1/1, Memory1/1
  Input/1 -> Sum1/1
  Memory1/1 -> Sum1/2

== system TestSetup/Uno#1: IPG//CPG Generating Arduino/Injection Signal Generator/Injection 3/Continuous Injection Signal Generator ==
  Input : Inport
  Reset : ResetPort  DisableCoverage=on
  Memory1 : Memory
  Sum1 : Sum  Inputs=|++
  Out1 : Outport
  wires:
  Sum1/1 -> Out1/1, Memory1/1
  Input/1 -> Sum1/1
  Memory1/1 -> Sum1/2

== system TestSetup/Uno#1: IPG//CPG Generating Arduino/Injection Signal Generator/Injection 4/Continuous Injection Signal Generator ==
  Input : Inport
  Reset : ResetPort  DisableCoverage=on
  Memory1 : Memory
  Sum1 : Sum  Inputs=|++
  Out1 : Outport
  wires:
  Sum1/1 -> Out1/1, Memory1/1
  Input/1 -> Sum1/1
  Memory1/1 -> Sum1/2
